simulink model "tarea"  (R2015a)
settings: Solver=ode45  StartTime=0.0  StopTime=10.0  RelTol=1e-3
settings Model: Creator=Alumnos  LastModifiedBy=Alumnos

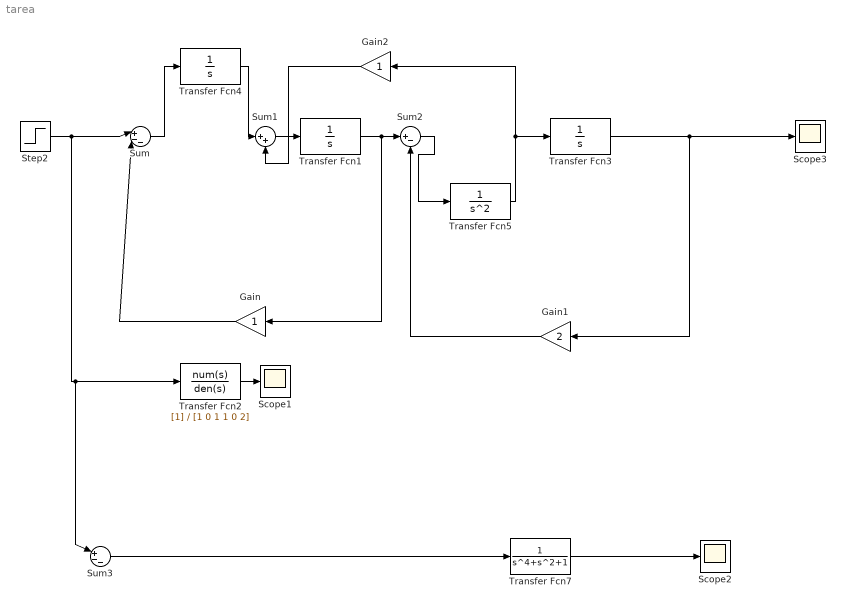
== system tarea ==
  Gain : Gain
  Gain1 : Gain  Gain=2
  Gain2 : Gain
  Scope1 : Scope
  Scope2 : Scope
      settings: SaveName=ScopeData2
  Scope3 : Scope
  Step2 : Step  SampleTime=0
  Sum : Sum  Inputs=|+--
  Sum1 : Sum  Inputs=|++
  Sum2 : Sum  Inputs=|+-
  Sum3 : Sum  Inputs=|+--
  Transfer Fcn1 : TransferFcn  Denominator=[1 0]
  Transfer Fcn2 : TransferFcn  Denominator=[1 0 1 1 0 2]
  Transfer Fcn3 : TransferFcn  Denominator=[1 0]
  Transfer Fcn4 : TransferFcn  Denominator=[1 0]
  Transfer Fcn5 : TransferFcn  Denominator=[1 0 0]
  Transfer Fcn7 : TransferFcn  Denominator=[1 0 1 0 1]
  wires:
  Gain/1 -> Sum/2
  Sum/1 -> Transfer Fcn4/1
  Transfer Fcn2/1 -> Scope1/1
  Transfer Fcn4/1 -> Sum1/1
  Sum1/1 -> Transfer Fcn1/1
  Transfer Fcn1/1 -> Gain/1, Sum2/1
  Transfer Fcn5/1 -> Gain2/1, Transfer Fcn3/1
  Transfer Fcn3/1 -> Gain1/1, Scope3/1
  Gain2/1 -> Sum1/2
  Sum2/1 -> Transfer Fcn5/1
  Gain1/1 -> Sum2/2
  Sum3/1 -> Transfer Fcn7/1
  Step2/1 -> Sum3/1, Transfer Fcn2/1, Sum/1
  Transfer Fcn7/1 -> Scope2/1
